simulink model "pm4_motor"  (R2017a)
settings: Solver=VariableStepAuto  StartTime=0.0  StopTime=3.0  RelTol=1e-3
libraries: simulink x1
settings Model: Creator=robotica  LastModifiedBy=robotica

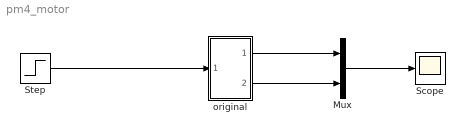
== system pm4_motor ==
  Mux : Mux  Inputs=2
  Scope : Scope
  Step : Step  SampleTime=1
  original : Subsystem
  wires:
  Step/1 -> original/1(signal)
  Mux/1 -> Scope/1
  original/1(noisy) -> Mux/1
  original/2(clean) -> Mux/2

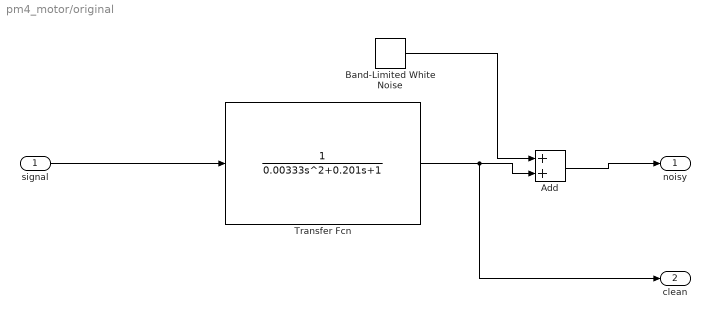
== system pm4_motor/original ==
  signal : Inport
  Add : Sum
  Band-Limited White Noise : simulink/Sources/Band-Limited White Noise  Cov=[0.0000001]  Ts=0.001  seed=[23341]
  Transfer Fcn : TransferFcn  Denominator=[0.00333 0.201 1]
  noisy : Outport
  clean : Outport  Port=2
  wires:
  Transfer Fcn/1 -> clean/1, Add/2
  Band-Limited White Noise/1 -> Add/1
  Add/1 -> noisy/1
  signal/1 -> Transfer Fcn/1
